simulink library "coordinate_transformations"  (R2019b)
settings: Solver=VariableStepAuto  StartTime=0.0  StopTime=10.0  RelTol=1e-3
settings Model: Creator=kissd  LastModifiedBy=kissd

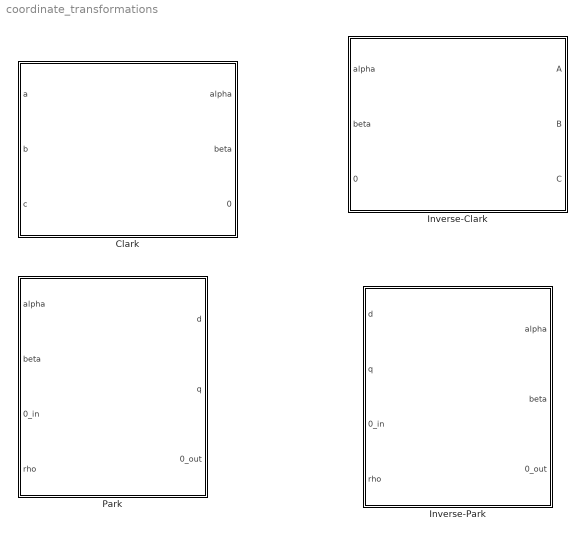
== system coordinate_transformations ==
  Clark : Subsystem
  Inverse-Clark : Subsystem
  Inverse-Park : Subsystem
  Park : Subsystem

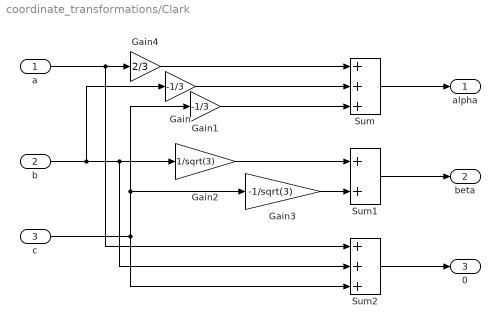
== system coordinate_transformations/Clark ==
  a : Inport
  b : Inport  Port=2
  c : Inport  Port=3
  Gain : Gain  Gain=-1/3
  Gain1 : Gain  Gain=-1/3
  Gain2 : Gain  Gain=1/sqrt(3)
  Gain3 : Gain  Gain=-1/sqrt(3)
  Gain4 : Gain  Gain=2/3
  Sum : Sum  Inputs=+++
  Sum1 : Sum
  Sum2 : Sum  Inputs=+++
  alpha : Outport
  beta : Outport  Port=2
  0 : Outport  Port=3
  wires:
  Sum/1 -> alpha/1
  a/1 -> Sum2/1, Gain4/1
  Gain/1 -> Sum/2
  Gain1/1 -> Sum/3
  b/1 -> Sum2/2, Gain2/1, Gain/1
  c/1 -> Gain3/1, Gain1/1, Sum2/3
  Sum1/1 -> beta/1
  Gain2/1 -> Sum1/1
  Gain3/1 -> Sum1/2
  Sum2/1 -> 0/1
  Gain4/1 -> Sum/1

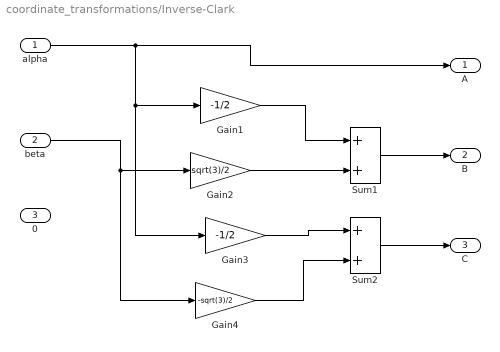
== system coordinate_transformations/Inverse-Clark ==
  alpha : Inport
  beta : Inport  Port=2
  0 : Inport  Port=3
  Gain1 : Gain  Gain=-1/2
  Gain2 : Gain  Gain=sqrt(3)/2
  Gain3 : Gain  Gain=-1/2
  Gain4 : Gain  Gain=-sqrt(3)/2
  Sum1 : Sum
  Sum2 : Sum
  A : Outport
  B : Outport  Port=2
  C : Outport  Port=3
  wires:
  alpha/1 -> Gain3/1, Gain1/1, A/1
  Sum1/1 -> B/1
  Gain2/1 -> Sum1/2
  Sum2/1 -> C/1
  Gain1/1 -> Sum1/1
  beta/1 -> Gain4/1, Gain2/1
  Gain3/1 -> Sum2/1
  Gain4/1 -> Sum2/2

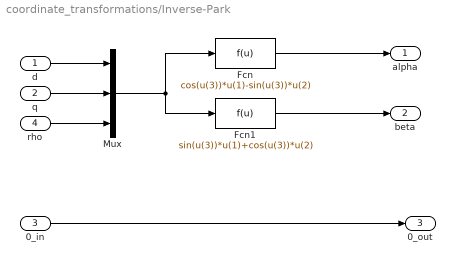
== system coordinate_transformations/Inverse-Park ==
  d : Inport
  q : Inport  Port=2
  0_in : Inport  Port=3
  rho : Inport  Port=4
  Fcn : Fcn  Expr=cos(u(3))*u(1)-sin(u(3))*u(2)
  Fcn1 : Fcn  Expr=sin(u(3))*u(1)+cos(u(3))*u(2)
  Mux : Mux  Inputs=3
  alpha : Outport
  beta : Outport  Port=2
  0_out : Outport  Port=3
  wires:
  0_in/1 -> 0_out/1
  Fcn/1 -> alpha/1
  Mux/1 -> Fcn1/1, Fcn/1
  q/1 -> Mux/2
  d/1 -> Mux/1
  rho/1 -> Mux/3
  Fcn1/1 -> beta/1

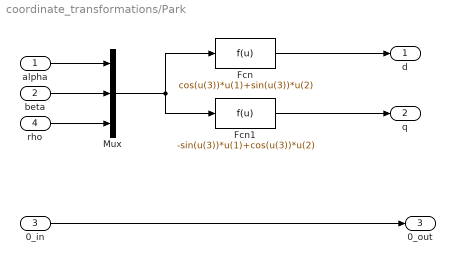
== system coordinate_transformations/Park ==
  alpha : Inport
  beta : Inport  Port=2
  0_in : Inport  Port=3
  rho : Inport  Port=4
  Fcn : Fcn  Expr=cos(u(3))*u(1)+sin(u(3))*u(2)
  Fcn1 : Fcn  Expr=-sin(u(3))*u(1)+cos(u(3))*u(2)
  Mux : Mux  Inputs=3
  d : Outport
  q : Outport  Port=2
  0_out : Outport  Port=3
  wires:
  0_in/1 -> 0_out/1
  Fcn/1 -> d/1
  Mux/1 -> Fcn1/1, Fcn/1
  beta/1 -> Mux/2
  alpha/1 -> Mux/1
  rho/1 -> Mux/3
  Fcn1/1 -> q/1
